simulink model "clik_phi_inverse"  (R2024b)
settings: Solver=ode1  StartTime=0.0  StopTime=4  FixedStep=0.001  RelTol=1e-3
undefined symbols (not defined in the file or in its folder): DiscIntNeverNeededParam, q0
settings Model: Creator=Xp  LastModifiedBy=22guo
settings SolverCC: AlgebraicLoopSolver=TrustRegion
settings DataIOCC: LimitDataPoints=on  SaveFormat=Array  SignalLoggingSaveFormat=ModelDataLogs  ReturnWorkspaceOutputs=off
settings OptimizationCC: ExpressionDepthLimit=2147483647  InitFltsAndDblsToZero=on  LifeSpan=inf
settings DebuggingCC: SaveWithParameterizedLinksMsg=none  UnderspecifiedInitializationDetection=Classic  MergeDetectMultiDrivingBlocksExec=none  SolverPrmCheckMsg=warning  MultiTaskDSMMsg=warning  MultiTaskCondExecSysMsg=none  FcnCallInpInsideContextMsg=warning  UnconnectedInputMsg=warning  UnconnectedOutputMsg=warning  UnconnectedLineMsg=warning  StateNameClashWarn=warning  SFUnexpectedBacktrackingDiag=warning  SFNoUnconditionalDefaultTransitionDiag=warning  SFExecutionAtInitializationDiag=none  ArithmeticOperatorsInVariantConditions=warning
settings HardwareCC: ProdBitPerPointer=32  ProdBitPerSizeT=32  ProdBitPerPtrDiffT=32  ProdLargestAtomicFloat=None  ProdIntDivRoundTo=Undefined  ProdEndianess=Unspecified  ProdWordSize=32  ProdHWDeviceType=32-bit Generic
settings ModelReferenceCC: EnableRefExpFcnMdlSchedulingChecks=on  PropagateSignalLabelsOutOfModel=off
settings SFSimCC: CustomCodeUndefinedFunction=UseInterfaceOnly
settings RTWCC: GPUComputeCapability=3.5  DLArmComputeVersion=19.05
settings CodeAppCC: StateflowObjectComments=on
settings GRTTargetCC: TargetLangStandard=C89/C90 (ANSI)  CombineOutputUpdateFcns=off  GRTInterface=on
settings ConfigComp: CovMetricSettings=dw  CovSaveCumulativeToWorkspaceVar=on  CovSaveSingleToWorkspaceVar=on

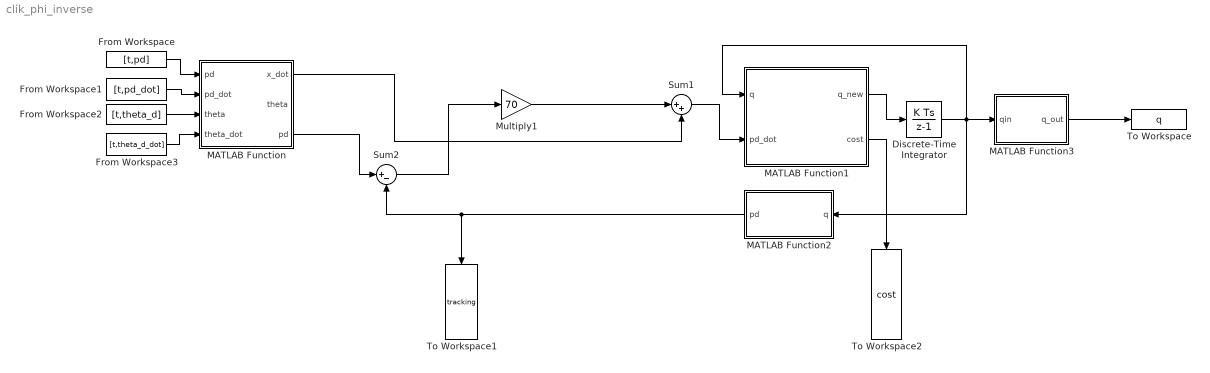
== system clik_phi_inverse ==
  Discrete-Time Integrator : DiscreteIntegrator  InitialCondition=q0(1:3)  SampleTime=0.001  ICPrevOutput=DiscIntNeverNeededParam  ICPrevScaledInput=DiscIntNeverNeededParam
  From Workspace : FromWorkspace  VariableName=[t,pd]  SampleTime=0.001
  From Workspace1 : FromWorkspace  VariableName=[t,pd_dot]  SampleTime=0.001
  From Workspace2 : FromWorkspace  VariableName=[t,theta_d]  SampleTime=0.001
  From Workspace3 : FromWorkspace  VariableName=[t,theta_d_dot]  SampleTime=0.001
  MATLAB Function : MATLAB Function  TreatAsAtomicUnit=on
  MATLAB Function1 : MATLAB Function  TreatAsAtomicUnit=on
  MATLAB Function2 : MATLAB Function  TreatAsAtomicUnit=on
  MATLAB Function3 : MATLAB Function  TreatAsAtomicUnit=on
  Multiply1 : Gain  Gain=70
  Sum1 : Sum  Inputs=|++
  Sum2 : Sum  Inputs=|+-
  To Workspace : ToWorkspace  VariableName=q  SampleTime=-1
  To Workspace1 : ToWorkspace  VariableName=tracking  SampleTime=-1
      settings: Save2DSignal=2-D array (concatenate along first dimension)
  To Workspace2 : ToWorkspace  VariableName=cost  SampleTime=-1
      settings: Save2DSignal=2-D array (concatenate along first dimension)
  wires:
  MATLAB Function2/1(pd) -> Sum2/2, To Workspace1/1
  Sum2/1 -> Multiply1/1
  MATLAB Function/3(pd) -> Sum2/1
  From Workspace2/1 -> MATLAB Function/3("theta ")
  Discrete-Time Integrator/1 -> MATLAB Function3/1(qin), MATLAB Function1/1(q), MATLAB Function2/1(q)
  MATLAB Function1/1(q_new) -> Discrete-Time Integrator/1
  From Workspace/1 -> MATLAB Function/1("pd ")
  MATLAB Function/1(x_dot) -> Sum1/2
  From Workspace3/1 -> MATLAB Function/4(theta_dot)
  Sum1/1 -> MATLAB Function1/2(pd_dot)
  Multiply1/1 -> Sum1/1
  From Workspace1/1 -> MATLAB Function/2(pd_dot)
  MATLAB Function1/2(cost) -> To Workspace2/1
  MATLAB Function3/1(q_out) -> To Workspace/1

== matlab function clik_phi_inverse/MATLAB Function1 ==
  data: q input; q_new output; pd_dot input; cost output
function [q_new, cost]= Psudo_inverse(q,pd_dot)
[q_new,cost]=jacobian_phi_relax(q,pd_dot);
end

== matlab function clik_phi_inverse/MATLAB Function ==
  data: pd input; pd_dot input; theta input; theta_dot input; x_dot output; theta output; pd output
function [x_dot,theta, pd]=data_prep(pd,pd_dot,theta,theta_dot)
pd=pd;
theta=theta;
x_dot=pd_dot';
end

== matlab function clik_phi_inverse/MATLAB Function2 ==
  data: q input; pd output
function pd = direct_k(q)
[pd] =direct_kin(q);
end

== matlab function clik_phi_inverse/MATLAB Function3 ==
  data: qin input; q_out output
function q_out = add_dim(qin)
q_out= [qin;0] %q4 is 0 since we relaxed it
end
